simulink model "audiosim"  (Simulink 7.0)
settings: Solver=FixedStepDiscrete  StartTime=0.0  StopTime=6.0  RelTol=1e-3
libraries: dspwin32 x1, simulink x1, dspsrcs4 x1, dspsnks4 x1, dspsigops x1
settings Model: Creator=dcs5  LastModifiedBy=dcs5

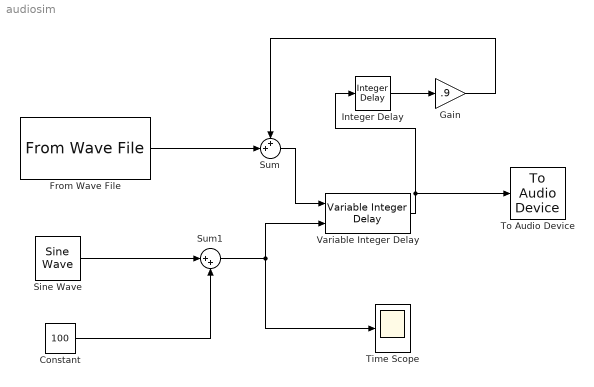
== system audiosim ==
  Constant : Constant  Value=100  OutDataType=sfix(16)  OutScaling=2^0  SampleTime=1/44100
      settings: SamplingMode=Frame based
  From Wave File : dspwin32/From Wave File  FileName=testing123dry.wav  SamplesPerFrame=1  MinBufSize=1  dType=double  bLoop=off  timesToPlay=1  restartMode=immediately after last sample  firstSampleOutput=off  lastSampleOutput=off
  Gain : Gain  Gain=.9  ParameterDataType=sfix(16)  ParameterScaling=2^0  OutDataType=sfix(16)  OutScaling=2^0
  Integer Delay : simulink/Discrete/Integer Delay  vinit=0  samptime=-1  NumDelays=100
  Sine Wave : dspsrcs4/Sine Wave  Amplitude=99  Frequency=.25  Phase=0  SampleMode=Discrete  OutComplex=Real  CompMethod=Trigonometric fcn  TableSize=Speed  SampleTime=1/44100  SamplesPerFrame=1  dataType=double  wordLen=16  udDataType=sfix(16)  fracBitsMode=Best precision  numFracBits=15  ResetState=Restart at time zero
  Sum : Sum  Inputs=++|  OutDataType=sfix(16)  OutScaling=2^0
  Sum1 : Sum  Inputs=|++  OutDataType=sfix(16)  OutScaling=2^0  SampleTime=1/44100
  Time Scope : Scope
      settings: TickLabels=on  TimeRange=6  YMin=0  YMax=200  DataFormat=Structure  Decimation=100
  To Audio Device : dspsnks4/To Audio Device  DialogController=dspDDGCreate  DialogControllerArgs=DataTag0  deviceName=Default  inheritSampleRate=on  sampleRate=44100  deviceDatatype=Determine from input data type  autoBufferSize=on  bufferSize=4096  queueDuration=1.0
  Variable Integer Delay : dspsigops/Variable Integer Delay  dmax=5000  ic=0
  wires:
  Constant/1 -> Sum1/2
  Sine Wave/1 -> Sum1/1
  Sum1/1 -> Variable Integer Delay/2, Time Scope/1
  Sum/1 -> Variable Integer Delay/1
  From Wave File/1 -> Sum/2
  Variable Integer Delay/1 -> Integer Delay/1, To Audio Device/1
  Integer Delay/1 -> Gain/1
  Gain/1 -> Sum/1
